simulink model "first_s_func2015"  (R2016a)
settings: Solver=VariableStepAuto  StartTime=0.0  StopTime=10.0  RelTol=1e-3
settings Model: Creator=DELL  LastModifiedBy=DELL
settings GRTTargetCC: GeneratePreprocessorConditionals=Use local settings
settings ConfigComp: CovModelRefEnable=Off

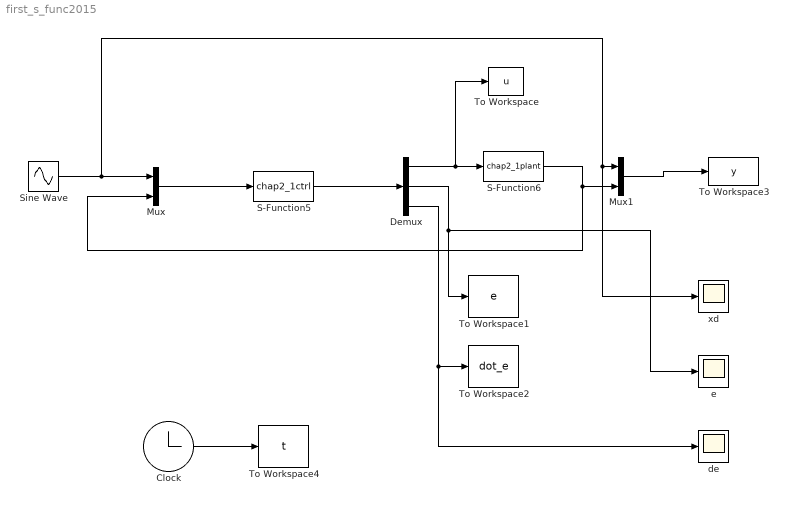
== system first_s_func2015 ==
  Clock : Clock
      settings: Decimation=15
  Demux : Demux  Outputs=3
  Mux : Mux  Inputs=2
  Mux1 : Mux  Inputs=2
  S-Function5 : S-Function  FunctionName=chap2_1ctrl  SFunctionDeploymentMode=off  EnableBusSupport=off
  S-Function6 : S-Function  FunctionName=chap2_1plant  SFunctionDeploymentMode=off  EnableBusSupport=off
  Sine Wave : Sin  SampleTime=0
  To Workspace : ToWorkspace  VariableName=u  SampleTime=-1
      settings: Save2DSignal=2-D array (concatenate along first dimension)
  To Workspace1 : ToWorkspace  VariableName=e  SampleTime=-1
      settings: Save2DSignal=2-D array (concatenate along first dimension)
  To Workspace2 : ToWorkspace  VariableName=dot_e  SampleTime=-1
      settings: Save2DSignal=2-D array (concatenate along first dimension)
  To Workspace3 : ToWorkspace  VariableName=y  SampleTime=-1
      settings: Save2DSignal=2-D array (concatenate along first dimension)
  To Workspace4 : ToWorkspace  VariableName=t  SampleTime=-1
      settings: Save2DSignal=2-D array (concatenate along first dimension)
  de : Scope
  e : Scope
  xd : Scope
  wires:
  Sine Wave/1 -> xd/1, Mux1/1, Mux/1
  S-Function5/1 -> Demux/1
  Demux/1 -> S-Function6/1, To Workspace/1
  Demux/2 -> e/1, To Workspace1/1
  Demux/3 -> de/1, To Workspace2/1
  S-Function6/1 -> Mux/2, Mux1/2
  Mux1/1 -> To Workspace3/1
  Clock/1 -> To Workspace4/1
  Mux/1 -> S-Function5/1
